simulink model "Cart_Pendulum_Linearised_b_9329013"  (R2017b)
settings: Solver=FixedStepAuto  StartTime=0.0  StopTime=10.0  FixedStep=0.05  RelTol=1e-3
values from neighbouring files (symbols this model uses):
  A = [0,0,1,0;0,0,0,1;0,((-m*g)/(Mc)),0,0;0,((g*(Mc+m))/(l*Mc)),0,0]    [CP_ContrSys_Lin_a_Mainfile_n9329013.m]    (also in CP_ContrSys_Lin_b_Mainfile_n9329013.m = [0,0,1,0;0,0,0,1;0,((-m*g)/(Mc)),0,0;0,-((g*(Mc+m))/(l*Mc)),; EGH445_Computer_Lab_1.m = [0,2,-8;3,5,4;-1.5,-1,1]; MainFile_Linearised_a_9329013.m; MainFile_Linearised_b_9329013.m = [0,0,1,0;0,0,0,1;0,((-m*g)/(Mc)),0,0;0,-((g*(Mc+m))/(l*Mc)),)
  B = [0,0,(1/Mc),-((1)/(l*Mc))]'    [CP_ContrSys_Lin_a_Mainfile_n9329013.m]    (also in CP_ContrSys_Lin_b_Mainfile_n9329013.m = [0,0,(1/Mc),((1)/(l*Mc))]'; EGH445_Computer_Lab_1.m = [4,4,0;1,4,0;-1,-2,2]; MainFile_Linearised_a_9329013.m; MainFile_Linearised_b_9329013.m = [0,0,(1/Mc),((1)/(l*Mc))]')
  C = eye(4)    [CP_ContrSys_Lin_a_Mainfile_n9329013.m]    (also in CP_ContrSys_Lin_b_Mainfile_n9329013.m; MainFile_Linearised_a_9329013.m; MainFile_Linearised_b_9329013.m)
  D = zeros(4,1)    [CP_ContrSys_Lin_a_Mainfile_n9329013.m]    (also in CP_ContrSys_Lin_b_Mainfile_n9329013.m; MainFile_Linearised_a_9329013.m; MainFile_Linearised_b_9329013.m)
settings Model: Creator=Koh Kim Hai  LastModifiedBy=Koh Kim Hai
settings DataIOCC: TimeSaveName=toutb_tilde

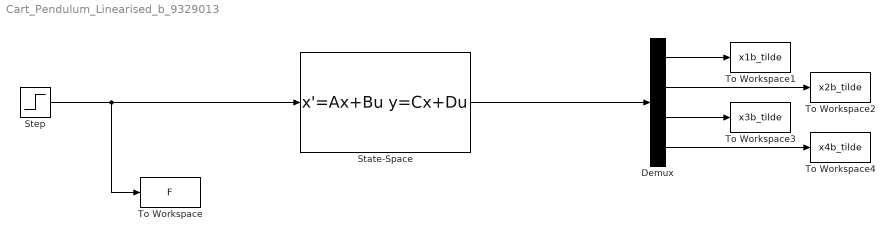
== system Cart_Pendulum_Linearised_b_9329013 ==
  Demux : Demux
  State-Space : StateSpace  A=A  B=B  C=C  D=D  InitialCondition=[0,pi,0,0]'
  Step : Step  After=0.1  SampleTime=0
  To Workspace : ToWorkspace  VariableName=F  SampleTime=-1
  To Workspace1 : ToWorkspace  VariableName=x1b_tilde  SampleTime=-1
  To Workspace2 : ToWorkspace  VariableName=x2b_tilde  SampleTime=-1
  To Workspace3 : ToWorkspace  VariableName=x3b_tilde  SampleTime=-1
  To Workspace4 : ToWorkspace  VariableName=x4b_tilde  SampleTime=-1
  wires:
  Step/1 -> To Workspace/1, State-Space/1
  State-Space/1 -> Demux/1
  Demux/2 -> To Workspace2/1
  Demux/3 -> To Workspace3/1
  Demux/4 -> To Workspace4/1
  Demux/1 -> To Workspace1/1
